simulink model "model_frac2"  (R2023a)
settings: Solver=VariableStepAuto  StartTime=0.0  StopTime=length(data)/100  RelTol=1e-3
values from neighbouring files (symbols this model uses):
  a = A(3)    [F1Vexp2V.m]    (also in F1Vexp2V_SexpS.m; F1Vexp2V_SexpS_ssr_all.m = input_parameters(3); F1Vexp3V.m; F1VexpV.m)
  alpha = input_parameters(1)    [Frac1Vexp2V_ssr.m]    (also in Frac1_ssr.m; Frac1_ssr_all.m = input_parameters(5); Frac1exp2V_ssr.m; Frac2_ssr.m)
  b = A(3)    [F1Sy.m]    (also in F1Vexp2V_SexpS.m = A(4); F1Vexp2V_SexpS_ssr.m = abs(b); F1Vexp2V_SexpS_ssr_all.m = input_parameters(5); F1VxSy.m = A(4))
  beta = input_parameters(2)    [Frac1Vexp2V_ssr.m]    (also in Frac1exp2V_ssr.m; Frac2_ssr.m)
  data = load(input_data)    [F1.m]    (also in F1Sy.m; F1Vexp2V.m; F1Vexp2V_SexpS.m; F1Vexp2V_SexpS_ssr.m)
  R = A(2)    [F1.m]    (also in F1Sy.m; F1Vexp2V.m; F1Vexp2V_SexpS.m; F1Vexp2V_SexpS_ssr_all.m = input_parameters(2))
libraries: voderiv x2
settings Model: Creator=test  LastModifiedBy=test

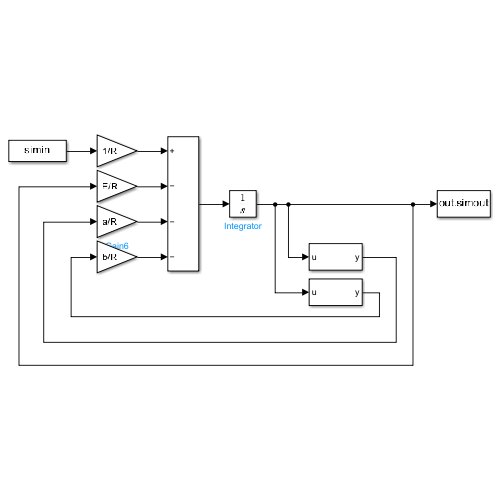
[thumbnail: Simulink's stored preview of the top-level diagram]
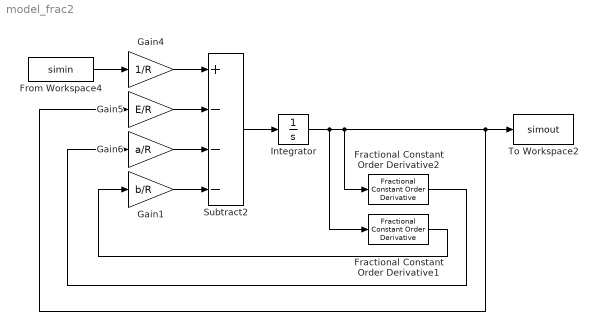
== system model_frac2 ==
  Fractional Constant Order Derivative1 : voderiv/Fractional Constant Order Derivative  N=beta  Nbuf=200  Ts=1
      settings: SourceProductName=Fractional Variable Order Derivative Toolkit III
  Fractional Constant Order Derivative2 : voderiv/Fractional Constant Order Derivative  N=alpha  Nbuf=200  Ts=1
      settings: SourceProductName=Fractional Variable Order Derivative Toolkit III
  From Workspace4 : FromWorkspace  VariableName=simin
  Gain1 : Gain  Gain=b/R
  Gain4 : Gain  Gain=1/R
  Gain5 : Gain  Gain=E/R
  Gain6 : Gain  Gain=a/R
  Integrator : Integrator  InitialCondition=data(1,3)
  Subtract2 : Sum  Inputs=+---
  To Workspace2 : ToWorkspace  VariableName=simout  SaveFormat=Timeseries  SampleTime=0.01
  wires:
  Fractional Constant Order Derivative2/1 -> Gain6/1
  Gain4/1 -> Subtract2/1
  Subtract2/1 -> Integrator/1
  Integrator/1 -> Fractional Constant Order Derivative1/1, To Workspace2/1, Gain5/1, Fractional Constant Order Derivative2/1
  Gain5/1 -> Subtract2/2
  From Workspace4/1 -> Gain4/1
  Gain6/1 -> Subtract2/3
  Gain1/1 -> Subtract2/4
  Fractional Constant Order Derivative1/1 -> Gain1/1
